simulink model "ControlArm"  (R2017a)
settings: Solver=VariableStepAuto  StartTime=0.0  StopTime=inf  RelTol=1e-3  EnableMultiTasking=on
undefined symbols (not defined in the file or in its folder): BodyIndexFrame, BodyTrackingID, ColorJointIndices, DepthJointIndices, HandLeftConfidence, HandLeftState, HandRightConfidence, HandRightState, IsBodyTracked, JointPositions, JointTrackingState, none, videoinput
libraries: imaqlib x1
settings Model: Creator=Bryan  LastModifiedBy=Bryan

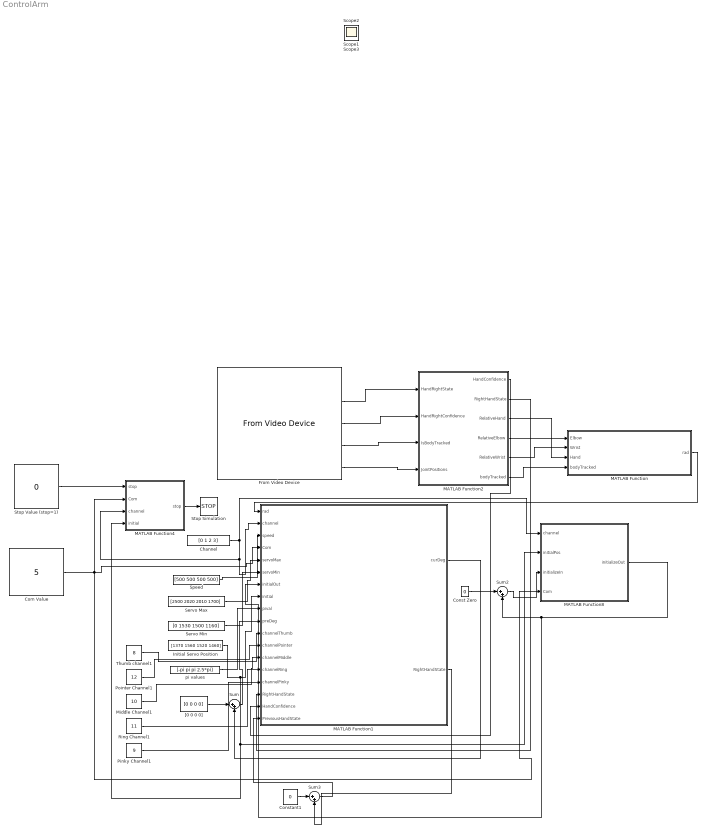
== system ControlArm ==
  Channel : Constant  Value=[0 1 2 3]
  Com Value : Constant  Value=5
  Const Zero : Constant  Value=0
  Constant1 : Constant  Value=0
  From Video Device : imaqlib/From Video Device  DeviceMenu=(none)  Device=kinect 2 (Kinect V2 Depth Sensor)  ObjConstructor=videoinput('kinect', 2)  VideoFormatMenu=(none)  VideoFormat=Depth_512x424  VideoSource=Kinect V2 Depth Source  ROIPosition=[0 0 424 512]  EnableHWTrigger=off  TriggerConfiguration=none/none  SampleTime=1/30  OutputPortsMode=One multidimensional signal  DataType=uint16  CanDoHWTrigger=no  ReturnedColorSpace=grayscale  BlockHandle=1823.0006  ROIWidth=512  ROIHeight=424  ROIColumn=0  ROIRow=0  EngXMLPath=C:\Program Files\MATLAB\R2017a\toolbox\imaq\imaq\private  DevXMLPath=C:\ProgramData\MATLAB\SupportPackages\R2017a\toolbox\imaq\supportpackages\kinectruntime\adaptor\win64  EngLibPath=C:\Program Files\MATLAB\R2017a\toolbox\imaq\imaqblks\imaqmex\win64  ColorSpace=grayscale  BayerSensorAlignment=grbg  AllMetadata=BodyIndexFrame;BodyTrackingID;ColorJointIndices;DepthJointIndices;HandLeftConfidence;HandLeftState;HandRightConfidence;HandRightState;IsBodyTracked;JointPositions;JointTrackingState  SelectedMetadata=HandRightState;HandRightConfidence;IsBodyTracked;JointPositions
      settings: SourceProductName=Image Acquisition Toolbox
  Initial Servo Position : Constant  Value=[1370 1560 1520 1460]
  MATLAB Function : MATLAB Function  TreatAsAtomicUnit=on
  MATLAB Function1 : MATLAB Function  TreatAsAtomicUnit=on
  MATLAB Function2 : MATLAB Function  TreatAsAtomicUnit=on
  MATLAB Function4 : MATLAB Function  TreatAsAtomicUnit=on
  MATLAB Function8 : MATLAB Function  TreatAsAtomicUnit=on
  Middle Channel1 : Constant  Value=10
  Pinky Channel1 : Constant  Value=9
  Pointer Channel1 : Constant  Value=12
  Ring Channel1 : Constant  Value=11
  Servo Max : Constant  Value=[2500 2020 2010 1700]
  Servo Min : Constant  Value=[0 1530 1500 1160]
  Speed : Constant  Value=[500 500 500 500]
  Stop Simulation : Stop
  Stop Value (stop=1) : Constant  Value=0
  Sum : Sum  Inputs=|++
  Sum2 : Sum  Inputs=|++
  Sum3 : Sum  Inputs=|++
  Thumb channel1 : Constant  Value=8
  "[0 0 0 0]" : Constant  Value=[0 0 0 0]
  pi values : Constant  Value=[-pi pi pi 2.5*pi]
  Scope1 : Scope
  Scope2 : Scope
  Scope3 : Scope
  wires:
  From Video Device/4 -> MATLAB Function2/3(IsBodyTracked)
  From Video Device/5 -> MATLAB Function2/4(JointPositions)
  From Video Device/3 -> MATLAB Function2/2(HandRightConfidence)
  From Video Device/2 -> MATLAB Function2/1(HandRightState)
  Sum2/1 -> MATLAB Function8/3(initializeIn)
  Const Zero/1 -> Sum2/1
  Com Value/1 -> MATLAB Function8/4(Com), MATLAB Function4/2(Com), MATLAB Function1/4(Com)
  MATLAB Function8/1(initializeOut) -> Sum2/2, MATLAB Function1/7(initialOut)
  MATLAB Function2/2(RightHandState) -> MATLAB Function1/16("RightHandState ")
  MATLAB Function2/1(HandConfidence) -> MATLAB Function1/17(HandConfidence)
  MATLAB Function2/6(bodyTracked) -> MATLAB Function/4(bodyTracked)
  MATLAB Function2/3(RelativeHand) -> MATLAB Function/3(Hand)
  MATLAB Function2/4(RelativeElbow) -> MATLAB Function/1(Elbow)
  MATLAB Function2/5(RelativeWrist) -> MATLAB Function/2(Wrist)
  Channel/1 -> MATLAB Function1/2(channel), MATLAB Function4/3(channel), MATLAB Function8/1(channel)
  Speed/1 -> MATLAB Function1/3(speed)
  Initial Servo Position/1 -> MATLAB Function4/4(initial), MATLAB Function8/2(initialPos), MATLAB Function1/8(initial)
  Sum/1 -> MATLAB Function1/10(preDeg)
  "[0 0 0 0]"/1 -> Sum/1
  MATLAB Function1/1(curDeg) -> Sum/2
  pi values/1 -> MATLAB Function1/9(pival)
  MATLAB Function/1(rad) -> MATLAB Function1/1(rad)
  MATLAB Function4/1(stop) -> Stop Simulation/1
  Stop Value (stop=1)/1 -> MATLAB Function4/1("stop ")
  Servo Max/1 -> MATLAB Function1/5(servoMax)
  Servo Min/1 -> MATLAB Function1/6(servoMin)
  Thumb channel1/1 -> MATLAB Function1/11(channelThumb)
  Pointer Channel1/1 -> MATLAB Function1/12(channelPointer)
  Middle Channel1/1 -> MATLAB Function1/13(channelMiddle)
  Ring Channel1/1 -> MATLAB Function1/14(channelRing)
  Pinky Channel1/1 -> MATLAB Function1/15(channelPinky)
  Constant1/1 -> Sum3/1
  Sum3/1 -> MATLAB Function1/18(PreviousHandState)
  MATLAB Function1/2(RightHandState) -> Sum3/2

== matlab function ControlArm/MATLAB Function ==
  data: rad output; Elbow input; Wrist input; Hand input; bodyTracked input

function rad  = jointAngles(Elbow, Wrist, Hand, bodyTracked)

    % This function takes in the Elbow, Wrist, and Hand joint positions
    % relative to the shoulder, and the bodyTracked condition. It calculates
    % the Shoulder1, Shoulder2, Elbow, and Wrist angles based on xyz
    % coordinates, and outputs a vector of joint angles in radians. 
    
    % If the body is not tracked, it outputs zero radians for all angles. 
    
    if bodyTracked == 0
        rad = [0 0 0 0];
    else

        wrist_rel = Wrist - Elbow;  %Calculate wrist xyz positions relative to elbow
        hand_rel = Hand - Wrist;    %Calculate hand xyz positions relative to wrist

        %Calculate shoulder1 angle 
        S1_angle = pi/2 + real(atan2(Elbow(2),Elbow(1)));
        if S1_angle > pi
            S1_angle = (2*pi - S1_angle)*(-1);    %Correct for direction of rotation
        end

        %Calcualte shoulder2 angle
        S2_angle = real(atan2(Elbow(3),sqrt(Elbow(1)^2+Elbow(2)^2)));

        %Calculate elbow angle
        E_angle = pi - real(acos(dot(Elbow/norm(Elbow), wrist_rel/norm(wrist_rel))));
        %Create forearm vector
        forearm = Wrist - Elbow; 
        %Create humerus vector 
        humerus = Elbow;   
        %Create normal vector of forerm-humerus 3D plane 
        normal = cross(forearm,humerus);    
        ratio = normal/hand_rel;
        if abs(ratio) > 1
            ratio = 1;     %Limit ratio
        end 
        
        %Calculate wrist angle
        W_angle = real(acos(real(ratio))) - pi/2;
        
        %If the wrist crosses the body 
        if Wrist(1) < 0
            W_angle = W_angle*(-1);
        end
        if W_angle < 0
            W_angle = W_angle*3;
        end
        
        %Concatinate radian vector
        rad = [S1_angle S2_angle E_angle W_angle];
        deg = [rad2deg(S1_angle) rad2deg(S2_angle) rad2deg(E_angle) rad2deg(W_angle)]
    end

== matlab function ControlArm/MATLAB Function4 ==
  data: stop input; stop output; Com input; channel input; initial input
function stop = fcn(stop, Com, channel, initial)
    
    % This function acts as stop for the Simulink simulation. If the stop
    % value is changed to 1, this function sends the arm back to its initial
    % position and ends the simulation. 
    
    % Please note: this function will not cut power to the servos.

    coder.extrinsic('serial','sprintf');

    if stop == 1
        formatCom='COM%d';
        format = '#%dP%d#%dP%d#%dP%d#%dP%dS500';
        ssc32 = serial(sprintf(formatCom,Com), 'BaudRate', 9600);
        set(ssc32,'Terminator','CR');
        fopen(ssc32);
        fprintf(ssc32,sprintf(format,channel(1),initial(1),channel(2), ...
                 initial(2),channel(3),initial(3),channel(4),initial(4)));
        fclose(ssc32);
    end

== matlab function ControlArm/MATLAB Function2 ==
  data: HandConfidence output; RightHandState output; HandRightState input; HandRightConfidence input; IsBodyTracked input; JointPositions input; RelativeHand output; RelativeElbow output; RelativeWrist output; bodyTracked output
function [HandConfidence,RightHandState,RelativeHand,RelativeElbow,RelativeWrist, bodyTracked] = kinectdata(...
                                                HandRightState,HandRightConfidence,IsBodyTracked,JointPositions)

    % This function takes in joint positions from the Kinect data and calculates vectors of hand, wrist, and elbow
    % positions relative to the shoulder position. It also ouputs a true/false if the body is sucessfully 
    % tracked or not, as well as hand state. 

    % Hand state vector: 0 unknown, 1 not tracked, 2 is open, 3 is closed, 4 is lasso
 
    %Find which index the body is being tracked in 
    BodyTracking = IsBodyTracked(:,:,1);
    for i = 1:1:length(BodyTracking)
        if BodyTracking(i) == 1
            index = i;
            break
        end
        index = i;
    end

    %Find if Kinect is tracking body or not
    bodyTracked = max(IsBodyTracked); % 1 = true

    %Calculate joint positions as xyz coordinates
    RightShoulderX = JointPositions(9,1,index);
    RightShoulderY = JointPositions(9,2,index);
    RightShoulderZ = JointPositions(9,3,index);
    Shoulder = [RightShoulderX,RightShoulderY,RightShoulderZ];

    RightElbowX = JointPositions(10,1,index);
    RightElbowY = JointPositions(10,2,index);
    RightElbowZ = JointPositions(10,3,index);

    RightWristX = JointPositions(11,1,index);
    RightWristY = JointPositions(11,2,index);
    RightWristZ = JointPositions(11,3,index);

    RightHandX = JointPositions(12,1,index);
    RightHandY = JointPositions(12,2,index);
    RightHandZ = JointPositions(12,3,index);

    RightHandTip = JointPositions(24,:,index);
    RightHandThumb = JointPositions(25,:,index);
    RightHandState = HandRightState(1,index); % Hand open, closed, or lasso
    HandConfidence = HandRightConfidence(1,index);

    %Calcualte positions relative to the shoulder (in xyz coordinates)
    RelativeHandX = RightHandX-RightShoulderX;
    RelativeHandY = RightHandY-RightShoulderY;
    RelativeHandZ = (RightHandZ-RightShoulderZ)*(-1); 
    RelativeHand = [RelativeHandX RelativeHandY RelativeHandZ]; %xyz coordinates

    RelativeElbowX = RightElbowX-RightShoulderX;
    RelativeElbowY = RightElbowY-RightShoulderY;
    RelativeEblowZ = (RightElbowZ-RightShoulderZ)*(-1);
    RelativeElbow = [RelativeElbowX RelativeElbowY RelativeEblowZ]; %xyz coordinates

    RelativeWristX = RightWristX-RightShoulderX;
    RelativeWristY = RightWristY-RightShoulderY;
    RelativeWristZ = (RightWristZ-RightShoulderZ)*(-1);
    RelativeWrist = [RelativeWristX RelativeWristY RelativeWristZ]; %xyz coordinates

== matlab function ControlArm/MATLAB Function8 ==
  data: channel input; initialPos input; initializeOut output; initializeIn input; Com input
function initializeOut = armInitialize(channel, initialPos, initializeIn, Com)
    
    % This function is the first move of the arm. It takes in the initial
    % servo positions of the arm, and sends the arm to those positions as a
    % starting point. Once the arm position is set, it outputs an
    % initializeOut flag of one. The rest of the code will not run until
    % this initialization is complete. 

    coder.extrinsic('serial','sprintf');    %Declare extrinsic function calls
        
    if initializeIn==0
        formatCom='COM%d';
        
        %Open servo connection 
        ssc32 = serial(sprintf(formatCom,Com), 'BaudRate', 9600);
        set(ssc32,'Terminator','CR');
        fopen(ssc32);
        speed=500;
        format='#%dP%dS%d';
        
        %Print to servos
        for i = 1:1:length(initialPos)
            fprintf(ssc32,sprintf(format,channel(i),initialPos(i),speed));
        end
        
        %Close servos
        fclose(ssc32);
        
    end
    
    %Set initialization flag to true
    initializeOut=1;

== matlab function ControlArm/MATLAB Function1 ==
  data: rad input; channel input; curDeg output; speed input; Com input; servoMax input; servoMin input; initialOut input; initial input; pival input; preDeg input; channelThumb input; channelPointer input; channelMiddle input; channelRing input; channelPinky input; RightHandState input; HandConfidence input; PreviousHandState input; RightHandState output
function [curDeg, RightHandState] = moveArm(rad, channel, speed, Com, servoMax, servoMin, initialOut, initial, pival, preDeg, ...
                            channelThumb, channelPointer, channelMiddle, channelRing, channelPinky, ...
                            RightHandState, HandConfidence, PreviousHandState)

     % This function takes in initial vectors for each servo and the vector
     % of radians of the wrist, elbow, and shoulder position. It takes the
     % radian information, converts it to degrees, and sends the joint to
     % the calculated degree if there was a detected degree change of more
     % than 0.5 deg. 
     
     % This function also puts limits on the servo output so that the arm 
     % does not damage itself or the base. 
   
     
     coder.extrinsic('serial','sprintf');
     
    if initialOut == 1     %If the initialization code has been completed
        
        %Initialize servo send
        formatCom='COM%d';
        ssc32 = serial(sprintf(formatCom,Com), 'BaudRate', 9600);
        set(ssc32,'Terminator','CR');
        fopen(ssc32);
        formatArm='#%fP%fS%d';
        
        %Hand movement code
        if HandConfidence==1 && PreviousHandState ~= RightHandState

             %Handcoded hand positions
             formatHand = '#%dP%dS500';
             thumbOpen=2050;
             thumbClose=1540;
             pointerOpen=1800;
             pointerClose=1070;
             middleOpen=1500;
             middleClose=780;
             ringOpen=960;
             ringClose=1660;
             pinkyOpen=1170;
             pinkyClose=2030;
             Speed=500;  %Constant speed for all channel  

             if RightHandState==2 %open hand      
                fprintf(ssc32,sprintf(formatHand,channelThumb,thumbOpen));
                fprintf(ssc32,sprintf(formatHand,channelPointer,pointerOpen));
                fprintf(ssc32,sprintf(formatHand,channelMiddle,middleOpen));
                fprintf(ssc32,sprintf(formatHand,channelRing,ringOpen));
                fprintf(ssc32,sprintf(formatHand,channelPinky,pinkyOpen));
             end
             if RightHandState==3 %closed hand
                fprintf(ssc32,sprintf(formatHand,channelThumb,thumbClose));
                fprintf(ssc32,sprintf(formatHand,channelPointer,pointerClose));
                fprintf(ssc32,sprintf(formatHand,channelMiddle,middleClose));
                fprintf(ssc32,sprintf(formatHand,channelRing,ringClose));
                fprintf(ssc32,sprintf(formatHand,channelPinky,pinkyClose));
             end  
             if RightHandState==4 %lasso
                fprintf(ssc32,sprintf(formatHand,channelThumb,thumbClose,channelPointer,pointerOpen,...
                channelMiddle,middleClose,channelRing,ringClose,channelPinky,pinkyOpen,Speed));
             end 
        end
        
        
        %Convert radians to degrees 
        curDeg = rad2deg(rad); %S1 S2 Elbow Wrist
        
        %For each joint, calculate servo position, test limits, and print
        %value to servos
        for i = 1:1:length(rad)
            if (abs(abs(curDeg(i))-abs(preDeg(i)))>0.5) %If a movement of greater than 0.5 deg is detected
                pos = initial(i) + curDeg(i)*pival(i);
                if pos > servoMax(i)                    %Upper limits
                    pos = servoMax(i);
                elseif pos < servoMin(i)                %Lower limits
                    pos = servoMin(i);
                end
                fprintf(ssc32,sprintf(formatArm,channel(i),pos,speed));  %Print to servos            
            end
        end
        
     
        %Close servo connection
        fclose(ssc32);
    else
        curDeg = [0 0 0 0];
    end
